simulink model "integrated_model_test"  (R2020a)
settings: Solver=FixedStepDiscrete  StartTime=0.0  StopTime=10.0  FixedStep=1  RelTol=1e-3
values from neighbouring files (symbols this model uses):
  Ignition : value not decoded    [ALS_Project_dd.sldd]
  Lanes : value not decoded    [ALS_Project_dd.sldd]
  Visual : value not decoded    [ALS_Project_dd.sldd]
undefined symbols (not defined in the file or in its folder): AlsMode, HeadLights, L1_max_distance, L1_min_distance, L2_max_distance, L2_min_distance, roads, speed
libraries: simulink x20
settings Model: DataDictionary=Als_dd.sldd  Creator=Pratik shinde  LastModifiedBy=Pratik shinde
settings OptimizationCC: DefaultParameterBehavior=Inlined  EnhancedBackFolding=on  PassReuseOutputArgsAs=Individual arguments  ZeroExternalMemoryAtStartup=off  ZeroInternalMemoryAtStartup=off  OptimizeBlockOrder=speed  DifferentSizesBufferReuse=on  OptimizationCustomize=off  EfficientTunableParamExpr=on
settings DebuggingCC: SignalInfNanChecking=error  SigSpecEnsureSampleTimeMsg=error  CheckMatrixSingularityMsg=error  IntegerOverflowMsg=error  ParameterTunabilityLossMsg=error  UnderSpecifiedDataTypeMsg=warning  UniqueDataStoreMsg=error  StrictBusMsg=ErrorOnBusTreatedAsVector  IntegerSaturationMsg=error
settings SFSimCC: MATLABDynamicMemAlloc=off
settings RTWCC: SystemTargetFile=ert.tlc  TemplateMakefile=ert_default_tmf
settings CodeAppCC: ForceParamTrailComments=on  IgnoreCustomStorageClasses=off  OperatorAnnotations=on  SimulinkDataObjDesc=on  SFDataObjDesc=on  InsertBlockDesc=on
settings ERTTargetCC: TargetLangStandard=C99 (ISO)  GenerateSampleERTMain=on  InlinedParameterPlacement=NonHierarchical  ERTCustomFileTemplate=example_file_process.tlc
settings ConfigComp: CovEnable=on  RecordCoverage=on  CovModelRefEnable=on  DVTestSuiteOptimization=Auto  DVDetectOutOfBounds=on

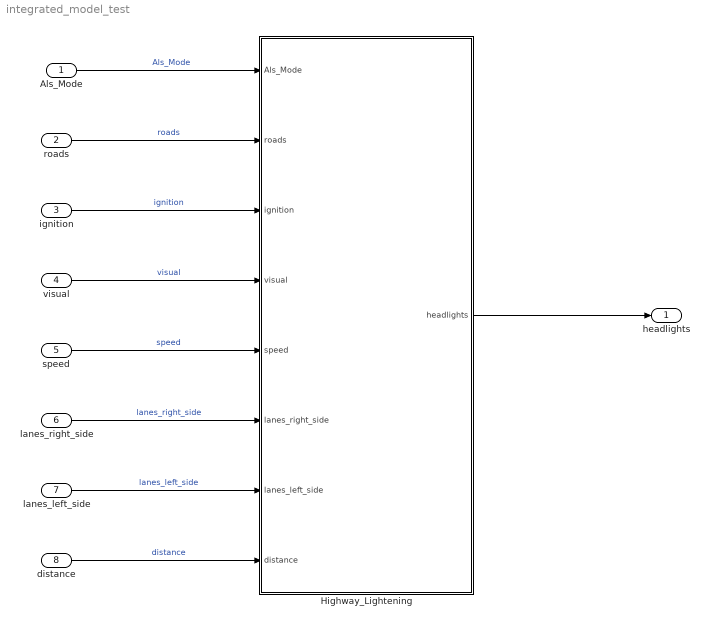
== system integrated_model_test ==
  Als_Mode : Inport
  roads : Inport  Port=2
  ignition : Inport  Port=3
  visual : Inport  Port=4
  speed : Inport  Port=5
  lanes_right_side : Inport  Port=6
  lanes_left_side : Inport  Port=7
  distance : Inport  Port=8
  Highway_Lightening : Subsystem  Description=this subsystem describes about the highway lightening system  TreatAsAtomicUnit=on
  headlights : Outport
  wires:
  lanes_left_side/1 -> Highway_Lightening/7(lanes_left_side)  "lanes_left_side"
  Highway_Lightening/1(headlights) -> headlights/1
  visual/1 -> Highway_Lightening/4(visual)  "visual"
  ignition/1 -> Highway_Lightening/3(ignition)  "ignition"
  lanes_right_side/1 -> Highway_Lightening/6(lanes_right_side)  "lanes_right_side"
  speed/1 -> Highway_Lightening/5(speed)  "speed"
  distance/1 -> Highway_Lightening/8(distance)  "distance"
  Als_Mode/1 -> Highway_Lightening/1(Als_Mode)  "Als_Mode"
  roads/1 -> Highway_Lightening/2(roads)  "roads"

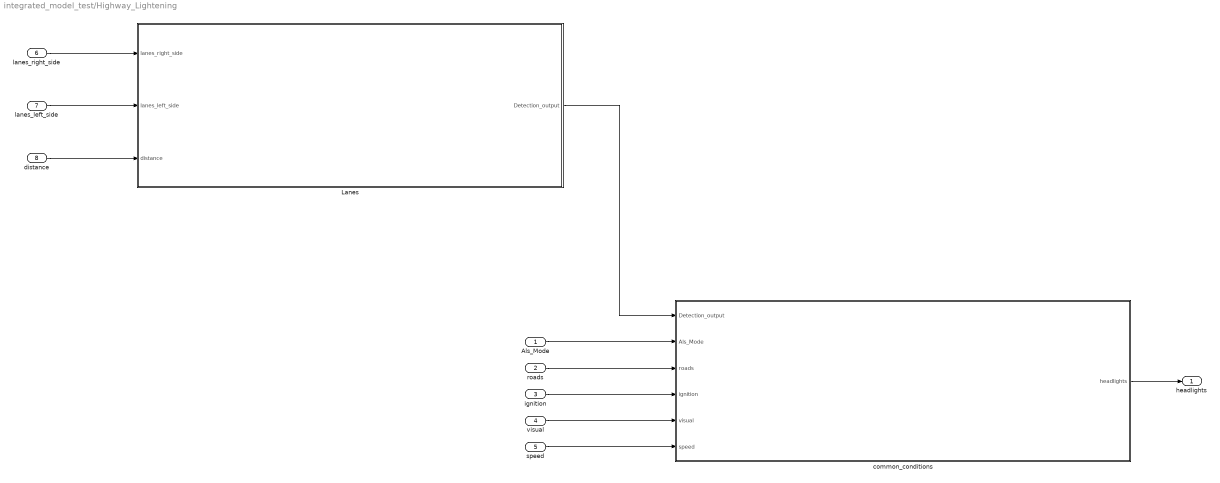
== system integrated_model_test/Highway_Lightening ==
  Als_Mode : Inport
  roads : Inport  Port=2
  ignition : Inport  Port=3
  visual : Inport  Port=4
  speed : Inport  Port=5
  lanes_right_side : Inport  Port=6
  lanes_left_side : Inport  Port=7
  distance : Inport  Port=8
  Lanes : Subsystem  Description=describes about the lanes scenario
  common_conditions : Subsystem  Description=normal lightening on highway
  headlights : Outport
  wires:
  lanes_right_side/1 -> Lanes/1(lanes_right_side)
  lanes_left_side/1 -> Lanes/2(lanes_left_side)
  distance/1 -> Lanes/3(distance)
  ignition/1 -> common_conditions/4(ignition)
  visual/1 -> common_conditions/5(visual)
  speed/1 -> common_conditions/6(speed)
  Lanes/1(Detection_output) -> common_conditions/1(Detection_output)
  Als_Mode/1 -> common_conditions/2(Als_Mode)
  roads/1 -> common_conditions/3(roads)
  common_conditions/1(headlights) -> headlights/1

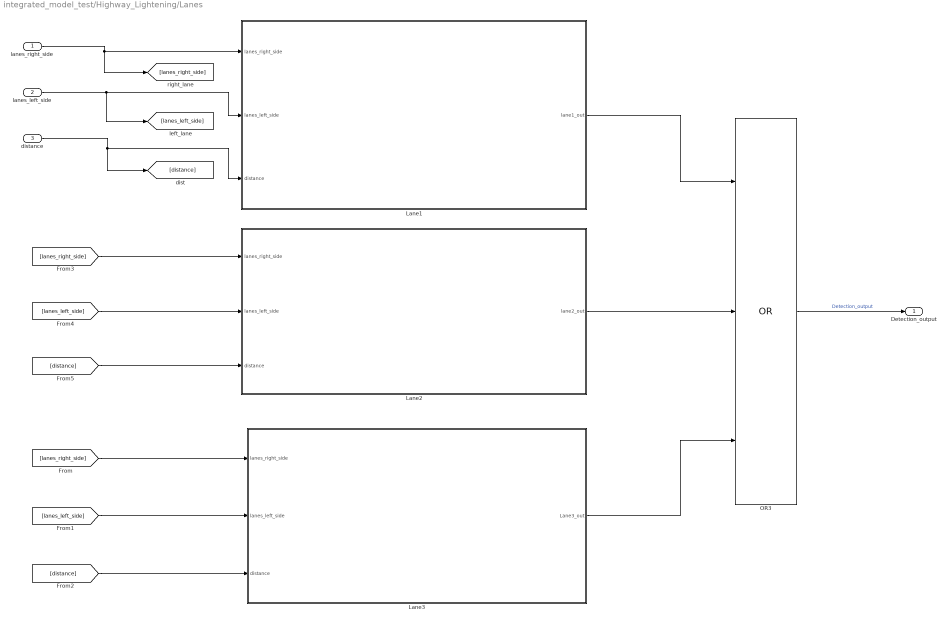
== system integrated_model_test/Highway_Lightening/Lanes ==
  lanes_right_side : Inport
  lanes_left_side : Inport  Port=2
  distance : Inport  Port=3
  Lane1 : Subsystem  Description=describes about the lane1 scenario
  Lane2 : Subsystem  Description=describes about the lane2 scenario
  Lane3 : Subsystem  Description=describes about the lane3 scenario
  OR3 : Logic  Operator=OR  Inputs=3  AllPortsSameDT=off  OutDataTypeStr=boolean
  Detection_output : Outport
  wires:
  Lane2/1(lane2_out) -> OR3/2
  Lane1/1(lane1_out) -> OR3/1
  Lane3/1(Lane3_out) -> OR3/3
  lanes_left_side/1 -> [lanes_left_side], Lane1/2(lanes_left_side)
  distance/1 -> [distance], Lane1/3(distance)
  lanes_right_side/1 -> [lanes_right_side], Lane1/1(lanes_right_side)
  [lanes_right_side] -> Lane3/1(lanes_right_side)
  [lanes_left_side] -> Lane3/2(lanes_left_side)
  [lanes_right_side] -> Lane2/1(lanes_right_side)
  [lanes_left_side] -> Lane2/2(lanes_left_side)
  [distance] -> Lane3/3(distance)
  [distance] -> Lane2/3(distance)
  OR3/1 -> Detection_output/1  "Detection_output"

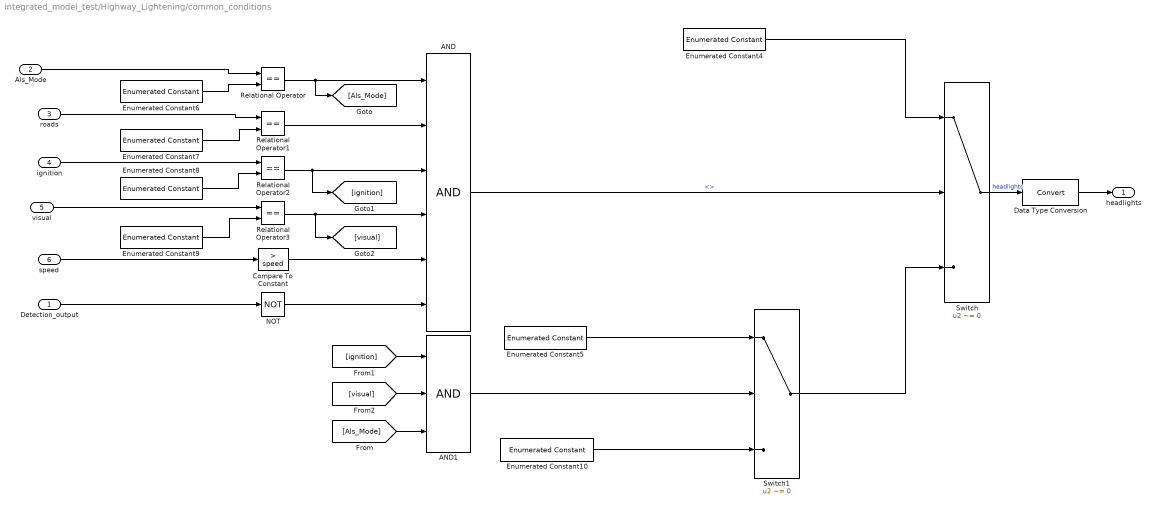
== system integrated_model_test/Highway_Lightening/common_conditions ==
  Detection_output : Inport
  Als_Mode : Inport  Port=2
  roads : Inport  Port=3
  ignition : Inport  Port=4
  visual : Inport  Port=5
  speed : Inport  Port=6
  AND : Logic  Inputs=6  AllPortsSameDT=off  OutDataTypeStr=boolean
  AND1 : Logic  Inputs=3  AllPortsSameDT=off  OutDataTypeStr=boolean
  Compare To Constant : simulink/Logic and Bit Operations/Compare To Constant  relop=>  const=speed  OutDataTypeStr=boolean
  Data Type Conversion : DataTypeConversion
  Enumerated Constant10 : simulink/Sources/Enumerated Constant  OutDataTypeStr=Enum:HeadLights  Value=HeadLights.HeadLight_Off  SampleTime=inf
  Enumerated Constant4 : simulink/Sources/Enumerated Constant  OutDataTypeStr=Enum: HeadLights  Value=HeadLights.HighBeam  SampleTime=inf
  Enumerated Constant5 : simulink/Sources/Enumerated Constant  OutDataTypeStr=Enum: HeadLights  Value=HeadLights.LowBeam  SampleTime=inf
  Enumerated Constant6 : simulink/Sources/Enumerated Constant  OutDataTypeStr=Enum: AlsMode  Value=AlsMode.On  SampleTime=inf
  Enumerated Constant7 : simulink/Sources/Enumerated Constant  OutDataTypeStr=Enum: roads  Value=roads.High_way  SampleTime=inf
  Enumerated Constant8 : simulink/Sources/Enumerated Constant  OutDataTypeStr=Enum: Ignition  Value=Ignition.On  SampleTime=inf
  Enumerated Constant9 : simulink/Sources/Enumerated Constant  OutDataTypeStr=Enum: Visual  Value=Visual.Night_Time  SampleTime=inf
  NOT : Logic  Operator=NOT  AllPortsSameDT=off  OutDataTypeStr=boolean
  Relational Operator{,1..3} (4 alike) : RelationalOperator  Operator===  OutDataTypeStr=boolean  RndMeth=Simplest
  Switch : Switch  Criteria=u2 ~= 0
  Switch1 : Switch  Criteria=u2 ~= 0
  headlights : Outport
  wires:
  Relational Operator3/1 -> [visual], AND/4
  Relational Operator/1 -> AND/1, [Als_Mode]
  Relational Operator2/1 -> [ignition], AND/3
  Enumerated Constant7/1 -> Relational Operator1/2
  Switch1/1 -> Switch/3
  AND1/1 -> Switch1/2
  Enumerated Constant9/1 -> Relational Operator3/2
  speed/1 -> Compare To Constant/1
  Compare To Constant/1 -> AND/5
  Als_Mode/1 -> Relational Operator/1
  roads/1 -> Relational Operator1/1
  AND/1 -> Switch/2  "<>"
  Enumerated Constant8/1 -> Relational Operator2/2
  ignition/1 -> Relational Operator2/1
  Switch/1 -> Data Type Conversion/1  "headlights"
  Relational Operator1/1 -> AND/2
  visual/1 -> Relational Operator3/1
  Detection_output/1 -> NOT/1
  Enumerated Constant6/1 -> Relational Operator/2
  NOT/1 -> AND/6
  [Als_Mode] -> AND1/3
  [ignition] -> AND1/1
  [visual] -> AND1/2
  Enumerated Constant4/1 -> Switch/1
  Enumerated Constant5/1 -> Switch1/1
  Enumerated Constant10/1 -> Switch1/3
  Data Type Conversion/1 -> headlights/1

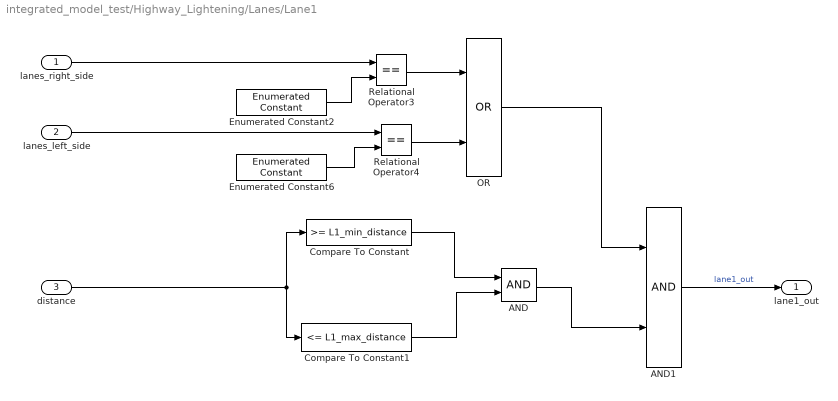
== system integrated_model_test/Highway_Lightening/Lanes/Lane1 ==
  lanes_right_side : Inport
  lanes_left_side : Inport  Port=2
  distance : Inport  Port=3
  AND : Logic  AllPortsSameDT=off  OutDataTypeStr=boolean
  AND1 : Logic  AllPortsSameDT=off  OutDataTypeStr=boolean
  Compare To Constant : simulink/Logic and Bit Operations/Compare To Constant  relop=>=  const=L1_min_distance  OutDataTypeStr=boolean
  Compare To Constant1 : simulink/Logic and Bit Operations/Compare To Constant  relop=<=  const=L1_max_distance  OutDataTypeStr=boolean
  Enumerated Constant2 : simulink/Sources/Enumerated Constant  OutDataTypeStr=Enum: Lanes  Value=Lanes.Lane1_right  SampleTime=inf
  Enumerated Constant6 : simulink/Sources/Enumerated Constant  OutDataTypeStr=Enum: Lanes  Value=Lanes.Lane1_left  SampleTime=inf
  OR : Logic  Operator=OR  AllPortsSameDT=off  OutDataTypeStr=boolean
  Relational Operator3 : RelationalOperator  Operator===  OutDataTypeStr=boolean  RndMeth=Simplest
  Relational Operator4 : RelationalOperator  Operator===  OutDataTypeStr=boolean  RndMeth=Simplest
  lane1_out : Outport
  wires:
  Enumerated Constant6/1 -> Relational Operator4/2
  Relational Operator3/1 -> OR/1
  Compare To Constant/1 -> AND/1
  OR/1 -> AND1/1
  distance/1 -> Compare To Constant/1, Compare To Constant1/1
  Enumerated Constant2/1 -> Relational Operator3/2
  lanes_left_side/1 -> Relational Operator4/1
  AND/1 -> AND1/2
  Compare To Constant1/1 -> AND/2
  Relational Operator4/1 -> OR/2
  lanes_right_side/1 -> Relational Operator3/1
  AND1/1 -> lane1_out/1  "lane1_out"

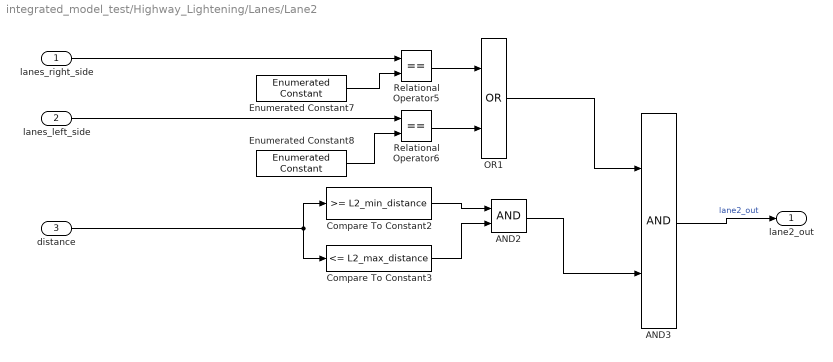
== system integrated_model_test/Highway_Lightening/Lanes/Lane2 ==
  lanes_right_side : Inport
  lanes_left_side : Inport  Port=2
  distance : Inport  Port=3
  AND2 : Logic  AllPortsSameDT=off  OutDataTypeStr=boolean
  AND3 : Logic  AllPortsSameDT=off  OutDataTypeStr=boolean
  Compare To Constant2 : simulink/Logic and Bit Operations/Compare To Constant  relop=>=  const=L2_min_distance  OutDataTypeStr=boolean
  Compare To Constant3 : simulink/Logic and Bit Operations/Compare To Constant  relop=<=  const=L2_max_distance  OutDataTypeStr=boolean
  Enumerated Constant7 : simulink/Sources/Enumerated Constant  OutDataTypeStr=Enum: Lanes  Value=Lanes.Lane2_right  SampleTime=inf
  Enumerated Constant8 : simulink/Sources/Enumerated Constant  OutDataTypeStr=Enum: Lanes  Value=Lanes.Lane2_left  SampleTime=inf
  OR1 : Logic  Operator=OR  AllPortsSameDT=off  OutDataTypeStr=boolean
  Relational Operator5 : RelationalOperator  Operator===  OutDataTypeStr=boolean  RndMeth=Simplest
  Relational Operator6 : RelationalOperator  Operator===  OutDataTypeStr=boolean  RndMeth=Simplest
  lane2_out : Outport
  wires:
  distance/1 -> Compare To Constant2/1, Compare To Constant3/1
  AND3/1 -> lane2_out/1  "lane2_out"
  lanes_left_side/1 -> Relational Operator6/1
  Compare To Constant3/1 -> AND2/2
  Enumerated Constant7/1 -> Relational Operator5/2
  OR1/1 -> AND3/1
  Compare To Constant2/1 -> AND2/1
  AND2/1 -> AND3/2
  Enumerated Constant8/1 -> Relational Operator6/2
  Relational Operator6/1 -> OR1/2
  Relational Operator5/1 -> OR1/1
  lanes_right_side/1 -> Relational Operator5/1

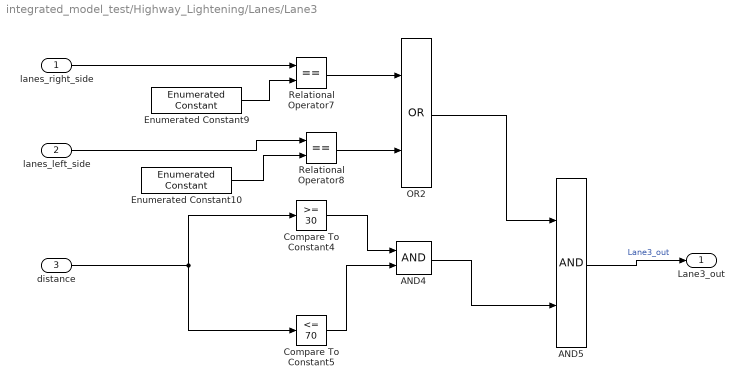
== system integrated_model_test/Highway_Lightening/Lanes/Lane3 ==
  lanes_right_side : Inport
  lanes_left_side : Inport  Port=2
  distance : Inport  Port=3
  AND4 : Logic  AllPortsSameDT=off  OutDataTypeStr=boolean
  AND5 : Logic  AllPortsSameDT=off  OutDataTypeStr=boolean
  Compare To Constant4 : simulink/Logic and Bit Operations/Compare To Constant  relop=>=  const=30  OutDataTypeStr=boolean
  Compare To Constant5 : simulink/Logic and Bit Operations/Compare To Constant  relop=<=  const=70  OutDataTypeStr=boolean
  Enumerated Constant10 : simulink/Sources/Enumerated Constant  OutDataTypeStr=Enum: Lanes  Value=Lanes.Lane3_left  SampleTime=inf
  Enumerated Constant9 : simulink/Sources/Enumerated Constant  OutDataTypeStr=Enum: Lanes  Value=Lanes.Lane3_right  SampleTime=inf
  OR2 : Logic  Operator=OR  AllPortsSameDT=off  OutDataTypeStr=boolean
  Relational Operator7 : RelationalOperator  Operator===  OutDataTypeStr=boolean  RndMeth=Simplest
  Relational Operator8 : RelationalOperator  Operator===  OutDataTypeStr=boolean  RndMeth=Simplest
  Lane3_out : Outport
  wires:
  distance/1 -> Compare To Constant4/1, Compare To Constant5/1
  Relational Operator8/1 -> OR2/2
  AND5/1 -> Lane3_out/1  "Lane3_out"
  Relational Operator7/1 -> OR2/1
  Compare To Constant5/1 -> AND4/2
  OR2/1 -> AND5/1
  Compare To Constant4/1 -> AND4/1
  AND4/1 -> AND5/2
  Enumerated Constant9/1 -> Relational Operator7/2
  Enumerated Constant10/1 -> Relational Operator8/2
  lanes_left_side/1 -> Relational Operator8/1
  lanes_right_side/1 -> Relational Operator7/1
